simulink model "DFIG_DTC_1"  (R2014a)
settings: Solver=ode23tb  StartTime=0.0  StopTime=1  RelTol=1e-3
libraries: powerlib x11, powerlib_meascontrol x5, simulink x1
settings Model: Creator=ninad gaikawad  LastModifiedBy=ninad gaikawad
settings SolverCC: ZeroCrossAlgorithm=Adaptive

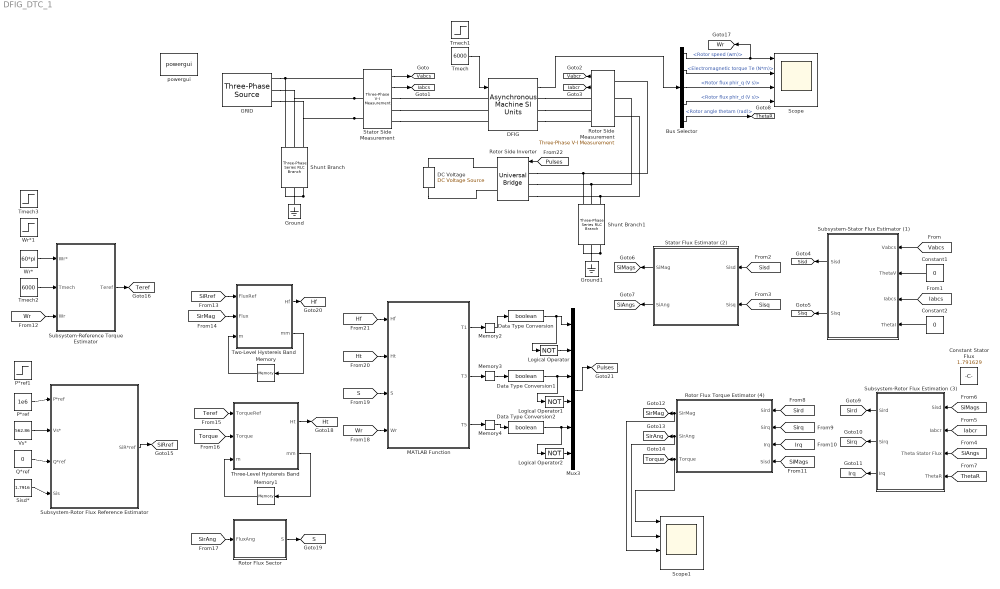
== system DFIG_DTC_1 ==
  Bus Selector : BusSelector  OutputSignals=Mechanical.Rotor speed (wm),Mechanical.Electromagnetic torque Te (N*m),Rotor measurements.Rotor flux phir_q (V s),Rotor measurements.Rotor flux phir_d (V s),Mechanical.Rotor angle thetam (rad)
  Constant Stator Flux : Constant  Value=1.791629
  Constant1 : Constant  Value=0
  Constant2 : Constant  Value=0
  DC Voltage : powerlib/Electrical Sources/DC Voltage Source  Amplitude=1200  Measurements=None
  DFIG : powerlib/Machines/Asynchronous Machine SI Units  PresetModel=No  MechanicalLoad=Torque Tm  ShowDetailedParameters=on  RotorType=Wound  ReferenceFrame=Rotor  Units=SI  MeasurementBus=off  NominalParameters=[1.5e+06 690 50]  Stator=[0.012 0.0137]  Rotor=[0.021 0.0136]  Cage1=[ 0.022 0.226/377]  Cage2=[ 0.022 0.226/377]  Lm=0.0135  Mechanical=[1000 30 2]  PolePairs=2  InitialConditions=[1 0 0 0 0 0 0 0]  SimulateSaturation=off  Saturation=[14.03593122, 27.81365428, 53.79336849, 72.68890987, 97.98006896, 148.6815601, 215.7428561, 302.9841135, 420.4778367 ; 230, 322, 414, 460, 506, 552, 598, 644, 690]  LoadFlowParameters=1492000  TsPowergui=0  TsBlock=-1  IterativeModel=Trapezoidal non iterative  Pmec=0
  Data Type Conversion : DataTypeConversion  OutDataTypeStr=boolean
  Data Type Conversion1 : DataTypeConversion  OutDataTypeStr=boolean
  Data Type Conversion2 : DataTypeConversion  OutDataTypeStr=boolean
  GRID : powerlib/Electrical Sources/Three-Phase Source  Voltage=25e3  PhaseAngle=0  Frequency=50  InternalConnection=Yg  SpecifyImpedance=off  Resistance=0  Inductance=0  ShortCircuitLevel=100e6  BaseVoltage=398  XRratio=7  BusType=swing  Pref=0  Qref=0  Qmin=-inf  Qmax=inf
  Ground : powerlib/Elements/Ground  LConnTagsString=a
  Ground1 : powerlib/Elements/Ground  LConnTagsString=a
  Logical Operator : Logic  Operator=NOT  AllPortsSameDT=off  OutDataTypeStr=boolean
  Logical Operator1 : Logic  Operator=NOT  AllPortsSameDT=off  OutDataTypeStr=boolean
  Logical Operator2 : Logic  Operator=NOT  AllPortsSameDT=off  OutDataTypeStr=boolean
  MATLAB Function : MATLAB Function  TreatAsAtomicUnit=on
  Memory : Memory  X0=1
  Memory1 : Memory  X0=1
  Memory2 : Memory  X0=1
  Memory3 : Memory
  Memory4 : Memory
  Mux3 : Mux  Inputs=6
  P*ref : Constant  Value=1e6
  P*ref1 : Step  Time=0.5  After=1e6  SampleTime=0
  Q*ref : Constant  Value=0
  Rotor Flux Sector : MATLAB Function  TreatAsAtomicUnit=on
  Rotor Flux Torque Estimator (4) : MATLAB Function  TreatAsAtomicUnit=on
  Rotor Side Inverter : powerlib/Power Electronics/Universal Bridge  Arms=3  SnubberResistance=1e5  SnubberCapacitance=inf  Device=IGBT / Diodes  Ron=1e-3  Lon=0  ForwardVoltages="[  0  0  ]"  ForwardVoltage=0  GTOparameters=[ 10e-6 , 20e-6 ]  IGBTparameters=[ 1e-6 , 2e-6 ]  Measurements=None  Measurements_2=None  converterType=Rectifier
  Rotor Side Measurement : powerlib/Measurements/Three-Phase V-I Measurement  VoltageMeasurement=phase-to-ground  SetLabelV=off  LabelV=Vabc  Vpu=off  VpuLL=off  CurrentMeasurement=yes  SetLabelI=off  LabelI=Iabc  Ipu=off  Pbase=100e6  Vbase=500e3  OutputType=Complex  PhasorSimulation=off  PSBequivalent=0
  Scope : Scope  NumInputPorts=4
      settings: YMin=-5~-5~-5~-5  YMax=5~5~5~5
  Scope1 : Scope  NumInputPorts=4
      settings: YMin=-5~-5~-5~-5  YMax=5~5~5~5
  Shunt Branch : powerlib/Elements/Three-Phase Series RLC Branch  LConnTagsString=A|B|C  RConnTagsString=A|B|C  BranchType=R  Resistance=1000  Inductance=1e-3  Capacitance=1e-6  Measurements=None
  Shunt Branch1 : powerlib/Elements/Three-Phase Series RLC Branch  LConnTagsString=A|B|C  RConnTagsString=A|B|C  BranchType=R  Resistance=10  Inductance=1e-3  Capacitance=1e-6  Measurements=None
  Sisd* : Constant  Value=1.7916
  Stator Flux Estimator (2) : MATLAB Function  TreatAsAtomicUnit=on
  Stator Side Measurement : powerlib/Measurements/Three-Phase V-I Measurement  VoltageMeasurement=phase-to-ground  SetLabelV=off  LabelV=Vabc  Vpu=off  VpuLL=off  CurrentMeasurement=yes  SetLabelI=off  LabelI=Iabc  Ipu=off  Pbase=100e6  Vbase=500e3  OutputType=Complex  PhasorSimulation=off  PSBequivalent=0
  Subsystem-Reference Torque Estimator : Subsystem
  Subsystem-Rotor Flux Estimation (3) : Subsystem
  Subsystem-Rotor Flux Reference Estimator : Subsystem
  Subsystem-Stator Flux Estimator (1) : Subsystem
  Three-Level Hystereis Band : MATLAB Function  TreatAsAtomicUnit=on
  Tmech : Constant  Value=6000
  Tmech1 : Step  Time=0.5  After=8000  SampleTime=0
  Tmech2 : Constant  Value=6000
  Tmech3 : Step  Time=0.5  After=8000  SampleTime=0
  Two-Level Hystereis Band : MATLAB Function  TreatAsAtomicUnit=on
  Vs* : Constant  Value=562.86
  Wr* : Constant  Value=60*pi
  Wr*1 : Step  Time=0.5  After=40*pi  SampleTime=0
  powergui : powerlib/powergui  Priority=1  SimulationMode=Continuous  SolverType=Tustin  SampleTime=50e-6  frequency=60  SPID=off  DisableSnubberDevices=off  DisableRonSwitches=off  DisableVfSwitches=off  SwTol=0  Interpol=off  DisplayEquations=off  Ts=0  methode=off  frequencyindice=50  Pbase=100e6  ErrMax=1e-4  Iterations=50  UnitsV=kV  UnitsW=MW  FunctionMessages=off  echomessages=off  HookPort=off  EnableUseOfTLC=off  x0status=blocks  RestoreLinks=warning  ResistiveCurrentMeasurement=off  Frange=[0:2:500]  Ylog=off  Xlog=on  ShowGrid=off  save=off  variable=ZData  structure=0  ZoomFFT=off  StartTime=0.0  cycles=1  DisplayStyle=1  fundamental=60  FreqAxis=off  MaxFrequency=1000  frequencyindicesteady=1  RmsSteady=1  display=off
  tag scope: Hf=global, Ht=global, Iabcr=global, Iabcs=global, Irq=global, Pulses=global, S=global, SiAngs=global, SiMags=global, SiRref=global, SirAng=global, SirMag=global, Sird=global, Sirq=global, Sisd=global, Sisq=global, Teref=global, ThetaR=global, Torque=global, Vabcr=global, Vabcs=global, Wr=global
  wires:
  DFIG/1 -> Bus Selector/1
  Stator Side Measurement/1 -> [Vabcs]
  Stator Side Measurement/2 -> [Iabcs]
  Rotor Side Measurement/1 -> [Vabcr]
  Rotor Side Measurement/2 -> [Iabcr]
  Bus Selector/2 -> Scope/2  "<Electromagnetic torque Te (N*m)>"
  Bus Selector/3 -> Scope/3  "<Rotor flux phir_q (V s)>"
  Bus Selector/4 -> Scope/4  "<Rotor flux phir_d (V s)>"
  Bus Selector/1 -> [Wr], Scope/1  "<Rotor speed (wm)>"
  [Vabcs] -> Subsystem-Stator Flux Estimator (1)/1(Vabcs)
  Constant1/1 -> Subsystem-Stator Flux Estimator (1)/2(ThetaV)
  [Iabcs] -> Subsystem-Stator Flux Estimator (1)/3(Iabcs)
  Constant2/1 -> Subsystem-Stator Flux Estimator (1)/4(ThetaI)
  Subsystem-Stator Flux Estimator (1)/1(Sisd) -> [Sisd]
  Subsystem-Stator Flux Estimator (1)/2(Sisq) -> [Sisq]
  [Sisd] -> Stator Flux Estimator (2)/1(Sisd)
  [Sisq] -> Stator Flux Estimator (2)/2(Sisq)
  Stator Flux Estimator (2)/2(SiAng) -> [SiAngs]
  Stator Flux Estimator (2)/1(SiMag) -> [SiMags]
  Bus Selector/5 -> [ThetaR]  "<Rotor angle thetam (rad)>"
  [SiMags] -> Subsystem-Rotor Flux Estimation (3)/1(Sisd)
  [Iabcr] -> Subsystem-Rotor Flux Estimation (3)/2(Iabcr)
  [SiAngs] -> Subsystem-Rotor Flux Estimation (3)/3(Theta Stator Flux)
  [ThetaR] -> Subsystem-Rotor Flux Estimation (3)/4(ThetaR)
  Subsystem-Rotor Flux Estimation (3)/2(Sirq) -> [Sirq]
  Subsystem-Rotor Flux Estimation (3)/1(Sird) -> [Sird]
  Subsystem-Rotor Flux Estimation (3)/3(Irq) -> [Irq]
  [SiMags] -> Rotor Flux Torque Estimator (4)/4(Sisd)
  [Irq] -> Rotor Flux Torque Estimator (4)/3(Irq)
  [Sirq] -> Rotor Flux Torque Estimator (4)/2(Sirq)
  [Sird] -> Rotor Flux Torque Estimator (4)/1(Sird)
  Rotor Flux Torque Estimator (4)/3(Torque) -> Scope1/1, [Torque]
  Q*ref/1 -> Subsystem-Rotor Flux Reference Estimator/3(Q*ref)
  Sisd*/1 -> Subsystem-Rotor Flux Reference Estimator/4(Sis)
  Subsystem-Rotor Flux Reference Estimator/1(SiR*ref) -> [SiRref]
  P*ref/1 -> Subsystem-Rotor Flux Reference Estimator/1(P*ref)
  Vs*/1 -> Subsystem-Rotor Flux Reference Estimator/2(Vs*)
  Tmech/1 -> DFIG/1
  Wr*/1 -> Subsystem-Reference Torque Estimator/1(Wr*)
  Subsystem-Reference Torque Estimator/1(Teref) -> [Teref]
  [Wr] -> Subsystem-Reference Torque Estimator/3(Wr)
  Tmech2/1 -> Subsystem-Reference Torque Estimator/2(Tmech)
  [SiRref] -> Two-Level Hystereis Band/1(FluxRef)
  [SirMag] -> Two-Level Hystereis Band/2(Flux)
  Two-Level Hystereis Band/2(mm) -> Memory/1
  Memory/1 -> Two-Level Hystereis Band/3(m)
  Three-Level Hystereis Band/2(mm) -> Memory1/1
  Memory1/1 -> Three-Level Hystereis Band/3(m)
  [Torque] -> Three-Level Hystereis Band/2(Torque)
  [Teref] -> Three-Level Hystereis Band/1(TorqueRef)
  [SirAng] -> Rotor Flux Sector/1(FluxAng)
  Rotor Flux Sector/1(S) -> [S]
  Three-Level Hystereis Band/1(Ht) -> [Ht]
  Two-Level Hystereis Band/1(Hf) -> [Hf]
  [Wr] -> MATLAB Function/4(Wr)
  Logical Operator1/1 -> Mux3/4
  Logical Operator/1 -> Mux3/2
  Logical Operator2/1 -> Mux3/6
  Data Type Conversion2/1 -> Logical Operator2/1, Mux3/5
  Data Type Conversion1/1 -> Logical Operator1/1, Mux3/3
  Memory2/1 -> Data Type Conversion/1
  MATLAB Function/1(T1) -> Memory2/1
  Memory3/1 -> Data Type Conversion1/1
  Memory4/1 -> Data Type Conversion2/1
  MATLAB Function/2(T3) -> Memory3/1
  MATLAB Function/3(T5) -> Memory4/1
  Data Type Conversion/1 -> Logical Operator/1, Mux3/1
  [Hf] -> MATLAB Function/1(Hf)
  [Ht] -> MATLAB Function/2(Ht)
  [S] -> MATLAB Function/3(S)
  Mux3/1 -> [Pulses]
  [Pulses] -> Rotor Side Inverter/1
  Rotor Flux Torque Estimator (4)/2(SirAng) -> Scope1/2, [SirAng]
  Rotor Flux Torque Estimator (4)/1(SirMag) -> Scope1/3, [SirMag]
  connections:
  GRID/RConn1 -- Stator Side Measurement/LConn1 -- Shunt Branch/LConn1
  Stator Side Measurement/LConn2 -- GRID/RConn2 -- Shunt Branch/LConn2
  Stator Side Measurement/LConn3 -- GRID/RConn3 -- Shunt Branch/LConn3
  Shunt Branch/RConn3 -- Shunt Branch/RConn1 -- Ground/LConn1 -- Shunt Branch/RConn2
  Rotor Side Inverter/LConn3 -- Shunt Branch1/LConn3 -- Rotor Side Measurement/LConn3
  DFIG/RConn2 -- Rotor Side Measurement/RConn2
  DFIG/RConn3 -- Rotor Side Measurement/RConn3
  Stator Side Measurement/RConn2 -- DFIG/LConn2
  Stator Side Measurement/RConn3 -- DFIG/LConn3
  Stator Side Measurement/RConn1 -- DFIG/LConn1
  DC Voltage/RConn1 -- Rotor Side Inverter/RConn1
  DC Voltage/LConn1 -- Rotor Side Inverter/RConn2
  DFIG/RConn1 -- Rotor Side Measurement/RConn1
  Rotor Side Inverter/LConn2 -- Shunt Branch1/LConn2 -- Rotor Side Measurement/LConn2
  Rotor Side Inverter/LConn1 -- Shunt Branch1/LConn1 -- Rotor Side Measurement/LConn1
  Shunt Branch1/RConn3 -- Shunt Branch1/RConn1 -- Ground1/LConn1 -- Shunt Branch1/RConn2

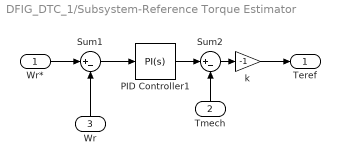
== system DFIG_DTC_1/Subsystem-Reference Torque Estimator ==
  Wr* : Inport
  Tmech : Inport  Port=2
  Wr : Inport  Port=3
  PID Controller1 : simulink/Continuous/PID Controller  Controller=PI  TimeDomain=Continuous-time  SampleTime=1  IntegratorMethod=Forward Euler  FilterMethod=Forward Euler  Form=Parallel  P=273.240186106265  I=55.6628456867696  D=0  N=100  InitialConditionSource=internal  InitialConditionForIntegrator=0  InitialConditionForFilter=0  ExternalReset=none  LimitOutput=off  UpperSaturationLimit=inf  LowerSaturationLimit=-inf  LinearizeAsGain=on  AntiWindupMode=none  Kb=1  TrackingMode=off  Kt=1  PParamMin=[]  PParamMax=[]  IParamMin=[]  IParamMax=[]  DParamMin=[]  DParamMax=[]  NParamMin=[]  NParamMax=[]  KbParamMin=[]  KbParamMax=[]  KtParamMin=[]  KtParamMax=[]  POutMin=[]  POutMax=[]  IOutMin=[]  IOutMax=[]  DOutMin=[]  DOutMax=[]  NOutMin=[]  NOutMax=[]  KbOutMin=[]  KbOutMax=[]  KtOutMin=[]  KtOutMax=[]  IntegratorOutMin=[]  IntegratorOutMax=[]  FilterOutMin=[]  FilterOutMax=[]  SumOutMin=[]  SumOutMax=[]  SumI1OutMin=[]  SumI1OutMax=[]  SumI2OutMin=[]  SumI2OutMax=[]  SumI3OutMin=[]  SumI3OutMax=[]  SumDOutMin=[]  SumDOutMax=[]  SaturationOutMin=[]  SaturationOutMax=[]  IntegratorContinuousStateAttributes=''  IntegratorStateMustResolveToSignalObject=off  IntegratorRTWStateStorageClass=Auto  FilterContinuousStateAttributes=''  FilterStateMustResolveToSignalObject=off  FilterRTWStateStorageClass=Auto
  Sum1 : Sum  Inputs=|+-
  Sum2 : Sum  Inputs=|+-
  k : Gain  Gain=-1
  Teref : Outport
  wires:
  Wr/1 -> Sum1/2
  Sum1/1 -> PID Controller1/1
  Tmech/1 -> Sum2/2
  PID Controller1/1 -> Sum2/1
  k/1 -> Teref/1
  Sum2/1 -> k/1
  Wr*/1 -> Sum1/1

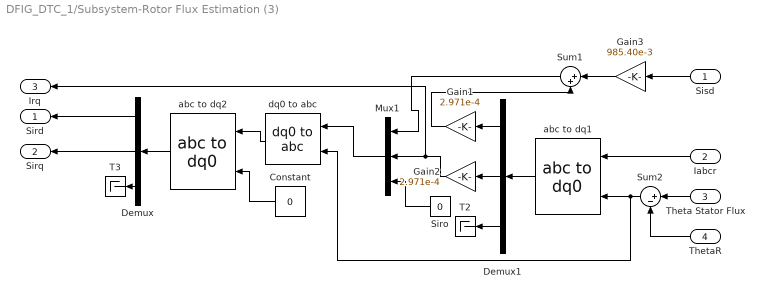
== system DFIG_DTC_1/Subsystem-Rotor Flux Estimation (3) ==
  Sisd : Inport
  Iabcr : Inport  Port=2
  Theta Stator Flux : Inport  Port=3
  ThetaR : Inport  Port=4
  Constant : Constant  Value=0
  Demux : Demux  Outputs=3
  Demux1 : Demux  Outputs=3
  Gain1 : Gain  Gain=2.971e-4
  Gain2 : Gain  Gain=2.971e-4
  Gain3 : Gain  Gain=985.40e-3
  Mux1 : Mux  Inputs=3
  Siro : Constant  Value=0
  Sum1 : Sum  Inputs=|++
  Sum2 : Sum  Inputs=|+-
  T2 : Terminator
  T3 : Terminator
  abc to dq1 : powerlib_meascontrol/Transformations/abc to dq0  Alignment=Aligned with phase A axis
  abc to dq2 : powerlib_meascontrol/Transformations/abc to dq0  Alignment=Aligned with phase A axis
  dq0 to abc : powerlib_meascontrol/Transformations/dq0 to abc  Alignment=Aligned with phase A axis
  Sird : Outport
  Sirq : Outport  Port=2
  Irq : Outport  Port=3
  wires:
  Sum1/1 -> Mux1/1
  Demux/3 -> T3/1
  Demux/2 -> Sirq/1
  Siro/1 -> Mux1/3
  Demux/1 -> Sird/1
  Iabcr/1 -> abc to dq1/1
  Gain1/1 -> Sum1/2
  Theta Stator Flux/1 -> Sum2/1
  Constant/1 -> abc to dq2/2
  Sum2/1 -> dq0 to abc/2, abc to dq1/2
  dq0 to abc/1 -> abc to dq2/1
  abc to dq2/1 -> Demux/1
  ThetaR/1 -> Sum2/2
  Demux1/1 -> Gain1/1
  Demux1/3 -> T2/1
  Demux1/2 -> Gain2/1
  abc to dq1/1 -> Demux1/1
  Mux1/1 -> dq0 to abc/1
  Gain2/1 -> Irq/1, Mux1/2
  Sisd/1 -> Gain3/1
  Gain3/1 -> Sum1/1

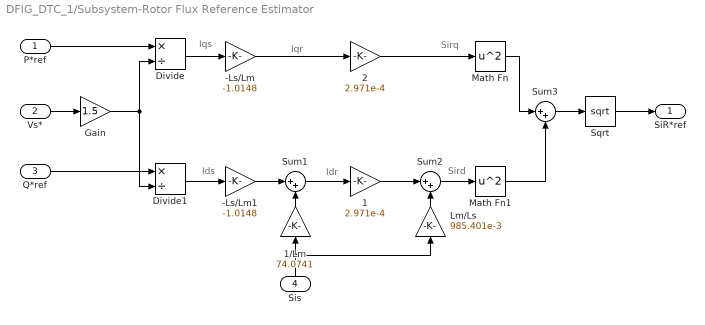
== system DFIG_DTC_1/Subsystem-Rotor Flux Reference Estimator ==
  note: Sird
  note: Sirq
  note: Ids
  note: Iqs
  note: Idr
  note: Iqr
  P*ref : Inport
  Vs* : Inport  Port=2
  Q*ref : Inport  Port=3
  Sis : Inport  Port=4
  -Ls/Lm : Gain  Gain=-1.0148
  -Ls/Lm1 : Gain  Gain=-1.0148
  1 : Gain  Gain=2.971e-4
  1/Lm : Gain  Gain=74.0741
  2 : Gain  Gain=2.971e-4
  Divide : Product  Inputs=*/
  Divide1 : Product  Inputs=*/
  Gain : Gain  Gain=1.5
  Lm/Ls : Gain  Gain=985.401e-3
  Math Fn : Math  Operator=square  SaturateOnIntegerOverflow=on
  Math Fn1 : Math  Operator=square  SaturateOnIntegerOverflow=on
  Sqrt : Sqrt  SaturateOnIntegerOverflow=on
  Sum1 : Sum  Inputs=|++
  Sum2 : Sum  Inputs=|++
  Sum3 : Sum  Inputs=|++
  SiR*ref : Outport
  wires:
  P*ref/1 -> Divide/1
  Vs*/1 -> Gain/1
  Q*ref/1 -> Divide1/1
  Divide/1 -> -Ls/Lm/1
  -Ls/Lm1/1 -> Sum1/1
  Sis/1 -> Lm/Ls/1, 1/Lm/1
  Divide1/1 -> -Ls/Lm1/1
  1/Lm/1 -> Sum1/2
  Gain/1 -> Divide1/2, Divide/2
  Sqrt/1 -> SiR*ref/1
  2/1 -> Math Fn/1
  1/1 -> Sum2/1
  Sum2/1 -> Math Fn1/1
  Sum1/1 -> 1/1
  -Ls/Lm/1 -> 2/1
  Math Fn1/1 -> Sum3/2
  Sum3/1 -> Sqrt/1
  Math Fn/1 -> Sum3/1
  Lm/Ls/1 -> Sum2/2

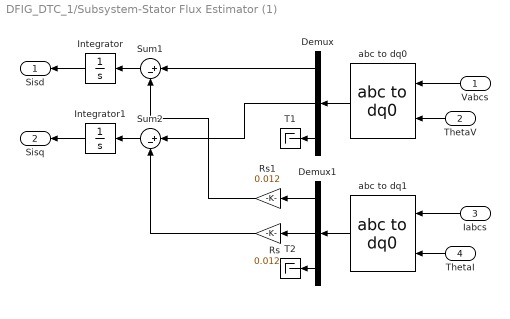
== system DFIG_DTC_1/Subsystem-Stator Flux Estimator (1) ==
  Vabcs : Inport
  ThetaV : Inport  Port=2
  Iabcs : Inport  Port=3
  ThetaI : Inport  Port=4
  Demux : Demux  Outputs=3
  Demux1 : Demux  Outputs=3
  Integrator : Integrator
  Integrator1 : Integrator
  Rs : Gain  Gain=0.012
  Rs1 : Gain  Gain=0.012
  Sum1 : Sum  Inputs=|+-
  Sum2 : Sum  Inputs=|+-
  T1 : Terminator
  T2 : Terminator
  abc to dq0 : powerlib_meascontrol/Transformations/abc to dq0  Alignment=Aligned with phase A axis
  abc to dq1 : powerlib_meascontrol/Transformations/abc to dq0  Alignment=Aligned with phase A axis
  Sisd : Outport
  Sisq : Outport  Port=2
  wires:
  Sum2/1 -> Integrator1/1
  Sum1/1 -> Integrator/1
  abc to dq0/1 -> Demux/1
  ThetaI/1 -> abc to dq1/2
  Iabcs/1 -> abc to dq1/1
  Rs1/1 -> Sum1/2
  Demux1/3 -> T2/1
  abc to dq1/1 -> Demux1/1
  Vabcs/1 -> abc to dq0/1
  Demux/1 -> Sum1/1
  Rs/1 -> Sum2/2
  Demux/3 -> T1/1
  Demux1/2 -> Rs/1
  Demux1/1 -> Rs1/1
  Demux/2 -> Sum2/1
  ThetaV/1 -> abc to dq0/2
  Integrator/1 -> Sisd/1
  Integrator1/1 -> Sisq/1

== matlab function DFIG_DTC_1/Two-Level Hystereis Band ==
  data: FluxRef input; Hf output; Flux input; m input; mm output
function [Hf,mm] = Two_Level_Hys(FluxRef,Flux,m)
 
DelF=0.025;% Hysteresis Width for Flux
Hf=0;%Initializing Hysteresis Controller Output For Flux
mm=m;
% Flux Two Level Hysteresis Band %
%------------------------------------------------------------------------%
if(Flux<=(FluxRef-DelF))
    Hf=1;
    mm=Hf;
end
if(mm==1&&(Flux>(FluxRef-DelF))&&(Flux<(FluxRef+DelF)))
    Hf=1;
    mm=Hf;
end
if(Flux>=(FluxRef+DelF))
    Hf=0;
    mm=Hf;
end
if(mm==0&&(Flux>(FluxRef-DelF))&&(Flux<(FluxRef+DelF)))
    Hf=0;
    mm=Hf;
end

== matlab function DFIG_DTC_1/Rotor Flux Torque Estimator (4) ==
  data: Sird input; SirMag output; Sirq input; Irq input; Sisd input; SirAng output; Torque output
function [SirMag,SirAng,Torque] = Rotor_Flux_Torque_Estimator(Sird,Sirq,Irq,Sisd)
 SirMag=((Sird)^(2)+(Sirq)^(2))^(0.5);
 x=atan2(Sirq,Sird);
 if(x>=0)
    SirAng=x*(180/pi);
 else
    SirAng=x*(180/pi)+360;
 end
 Torque=(-3)*(0.0135/0.0136)*(Sisd*Irq);

== matlab function DFIG_DTC_1/Stator Flux Estimator (2) ==
  settings: updateMethod=CONTINUOUS
  data: Sisd input; SiMag output; Sisq input; SiAng output
function [SiMag,SiAng] = StatorFlux_MagAng_Estimator(Sisd,Sisq)
 SiMag=((Sisd)^(2)+(Sisq)^(2))^(0.5);
 x=atan2(Sisq,Sisd);
 if(x>=0)
    SiAng=x;
 else
    SiAng=x+(2*pi);
 end

== matlab function DFIG_DTC_1/Three-Level Hystereis Band ==
  data: TorqueRef input; Ht output; Torque input; m input; mm output
function [Ht,mm] = Three_Level_Hys(TorqueRef,Torque,m)
 
DelT=1;% Hysteresis Width for Torque
Ht=0;%Initializing Hysteresis Controller Output For Torque
mm=m;

% Torque Three Level Hysteresis Band %
%------------------------------------------------------------------------%
if(Torque<=(TorqueRef-DelT))
    Ht=1;
    mm=Ht;
end
if((Torque>(TorqueRef-DelT))&&(Torque<TorqueRef)&&mm==1)
    Ht=1;
    mm=Ht;
end
if(Torque>=(TorqueRef+DelT))
    Ht=-1;
    mm=Ht;
end
if((Torque<(TorqueRef+DelT))&&(Torque>TorqueRef)&&mm==-1)
    Ht=-1;
    mm=Ht;
end
if((Torque>(TorqueRef-DelT))&&(Torque<TorqueRef)&&mm==-1)
    Ht=0;
    mm=-1;
end
if((Torque<(TorqueRef+DelT))&&(Torque>TorqueRef)&&mm==1)
    Ht=0;
    mm=1;
end

== matlab function DFIG_DTC_1/Rotor Flux Sector ==
  data: FluxAng input; S output
function S= Rotor_Flux_Sector(FluxAng)
 

% DTC Sector Prediction %
%------------------------------------------------------------------------%
if(FluxAng>=330&&FluxAng<30)
    S=1;
end
if(FluxAng>=30&&FluxAng<90)
    S=2;
end
if(FluxAng>=90&&FluxAng<150)
    S=3;
end
if(FluxAng>=150&&FluxAng<210)
    S=4;
end
if(FluxAng>=210&&FluxAng<270)
    S=5;
end
if(FluxAng>=270&&FluxAng<330)
    S=6;
end

== matlab function DFIG_DTC_1/MATLAB Function ==
  data: Hf input; T1 output; Ht input; S input; Wr input; T3 output; T5 output
function [T1,T3,T5] = DTC_SwitchingTable(Hf,Ht,S,Wr)
 
T1=0;
T3=0;
T5=0;

% Voltage Vector Synthesis %
%------------------------------------------------------------------------%
if(Wr<=(50*pi))% Sub-Synchronous
%------------------------------------------------------------------------%    
    if(Hf==1&&Ht==1&&S==1)
        T1=1;
        T3=0;
        T5=1;
    end
    if(Hf==1&&Ht==1&&S==2)
      T1=0;
      T3=0;
      T5=1;  
    end
    if(Hf==1&&Ht==1&&S==3)
      T1=0;
      T3=1;
      T5=1; 
    end
    if(Hf==1&&Ht==1&&S==4)
      T1=0;
      T3=1;
      T5=0;
    end
    if(Hf==1&&Ht==1&&S==5)
      T1=1;
      T3=1;
      T5=0;    
    end
    if(Hf==1&&Ht==1&&S==6)
      T1=1;
      T3=0;
      T5=0;
    end
   
%------------------------------------------------------------------------%    
    if(Hf==1&&Ht==0&&S==1)
        T1=1;
        T3=1;
        T5=1;
    end
    if(Hf==1&&Ht==0&&S==2)
      T1=0;
      T3=0;
      T5=0;  
    end
    if(Hf==1&&Ht==0&&S==3)
      T1=1;
      T3=1;
      T5=1; 
    end
    if(Hf==1&&Ht==0&&S==4)
      T1=0;
      T3=0;
      T5=0;
    end
    if(Hf==1&&Ht==0&&S==5)
      T1=1;
      T3=1;
      T5=1;    
    end
    if(Hf==1&&Ht==0&&S==6)
      T1=0;
      T3=0;
      T5=0;
    end
%------------------------------------------------------------------------%    
    if(Hf==1&&Ht==-1&&S==1)
        T1=1;
        T3=1;
        T5=0;
    end
    if(Hf==1&&Ht==-1&&S==2)
      T1=1;
      T3=0;
      T5=0;  
    end
    if(Hf==1&&Ht==-1&&S==3)
      T1=1;
      T3=0;
      T5=1; 
    end
    if(Hf==1&&Ht==-1&&S==4)
      T1=0;
      T3=0;
      T5=1;
    end
    if(Hf==1&&Ht==-1&&S==5)
      T1=0;
      T3=1;
      T5=1;    
    end
    if(Hf==1&&Ht==-1&&S==6)
      T1=0;
      T3=1;
      T5=0;
    end
    
 %------------------------------------------------------------------------%   
    
     if(Hf==0&&Ht==1&&S==1)
        T1=0;
        T3=0;
        T5=1;
    end
    if(Hf==0&&Ht==1&&S==2)
      T1=0;
      T3=1;
      T5=1;  
    end
    if(Hf==0&&Ht==1&&S==3)
      T1=0;
      T3=1;
      T5=0; 
    end
    if(Hf==0&&Ht==1&&S==4)
      T1=1;
      T3=1;
      T5=0;
    end
    if(Hf==0&&Ht==1&&S==5)
      T1=1;
      T3=0;
      T5=0;    
    end
    if(Hf==0&&Ht==1&&S==6)
      T1=1;
      T3=0;
      T5=1;
    end
%------------------------------------------------------------------------%    
    
    if(Hf==0&&Ht==0&&S==1)
        T1=0;
        T3=0;
        T5=0;
    end
    if(Hf==0&&Ht==0&&S==2)
      T1=1;
      T3=1;
      T5=1;  
    end
    if(Hf==0&&Ht==0&&S==3)
      T1=0;
      T3=0;
      T5=0; 
    end
    if(Hf==0&&Ht==0&&S==4)
      T1=1;
      T3=1;
      T5=1;
    end
    if(Hf==0&&Ht==0&&S==5)
      T1=0;
      T3=0;
      T5=0;    
    end
    if(Hf==0&&Ht==0&&S==6)
      T1=1;
      T3=1;
      T5=1;
    end
  %------------------------------------------------------------------------%  
    
    if(Hf==0&&Ht==-1&&S==1)
        T1=0;
        T3=1;
        T5=0;
    end
    if(Hf==0&&Ht==-1&&S==2)
      T1=1;
      T3=1;
      T5=0;  
    end
    if(Hf==0&&Ht==-1&&S==3)
      T1=1;
      T3=0;
      T5=0; 
    end
    if(Hf==0&&Ht==-1&&S==4)
      T1=1;
      T3=0;
      T5=1;
    end
    if(Hf==0&&Ht==-1&&S==5)
      T1=0;
      T3=0;
      T5=1;    
    end
    if(Hf==0&&Ht==-1&&S==6)
      T1=0;
      T3=1;
      T5=1;
    end
end

%------------------------------------------------------------------------%
if(Wr>(50*pi))% Super-Synchronous
%------------------------------------------------------------------------%    
    if(Hf==1&&Ht==1&&S==1)
        T1=1;
        T3=0;
        T5=1;
    end
    if(Hf==1&&Ht==1&&S==2)
      T1=1;
      T3=0;
      T5=0;  
    end
    if(Hf==1&&Ht==1&&S==3)
      T1=1;
      T3=1;
      T5=0; 
    end
    if(Hf==1&&Ht==1&&S==4)
      T1=0;
      T3=1;
      T5=0;
    end
    if(Hf==1&&Ht==1&&S==5)
      T1=0;
      T3=1;
      T5=1;    
    end
    if(Hf==1&&Ht==1&&S==6)
      T1=0;
      T3=0;
      T5=1;
    end
   
%------------------------------------------------------------------------%    
    if(Hf==1&&Ht==0&&S==1)
        T1=1;
        T3=1;
        T5=1;
    end
    if(Hf==1&&Ht==0&&S==2)
      T1=0;
      T3=0;
      T5=0;  
    end
    if(Hf==1&&Ht==0&&S==3)
      T1=1;
      T3=1;
      T5=1; 
    end
    if(Hf==1&&Ht==0&&S==4)
      T1=0;
      T3=0;
      T5=0;
    end
    if(Hf==1&&Ht==0&&S==5)
      T1=1;
      T3=1;
      T5=1;    
    end
    if(Hf==1&&Ht==0&&S==6)
      T1=0;
      T3=0;
      T5=0;
    end
%------------------------------------------------------------------------%    
    if(Hf==1&&Ht==-1&&S==1)
        T1=1;
        T3=0;
        T5=0;
    end
    if(Hf==1&&Ht==-1&&S==2)
      T1=1;
      T3=1;
      T5=0;  
    end
    if(Hf==1&&Ht==-1&&S==3)
      T1=0;
      T3=1;
      T5=0; 
    end
    if(Hf==1&&Ht==-1&&S==4)
      T1=0;
      T3=1;
      T5=1;
    end
    if(Hf==1&&Ht==-1&&S==5)
      T1=0;
      T3=0;
      T5=1;    
    end
    if(Hf==1&&Ht==-1&&S==6)
      T1=1;
      T3=0;
      T5=1;
    end
    
 %------------------------------------------------------------------------%   
    
     if(Hf==0&&Ht==1&&S==1)
        T1=0;
        T3=0;
        T5=1;
    end
    if(Hf==0&&Ht==1&&S==2)
      T1=1;
      T3=0;
      T5=1;  
    end
    if(Hf==0&&Ht==1&&S==3)
      T1=1;
      T3=0;
      T5=0; 
    end
    if(Hf==0&&Ht==1&&S==4)
      T1=1;
      T3=1;
      T5=0;
    end
    if(Hf==0&&Ht==1&&S==5)
      T1=0;
      T3=1;
      T5=0;    
    end
    if(Hf==0&&Ht==1&&S==6)
      T1=0;
      T3=1;
      T5=1;
    end
%------------------------------------------------------------------------%    
    
    if(Hf==0&&Ht==0&&S==1)
        T1=0;
        T3=0;
        T5=0;
    end
    if(Hf==0&&Ht==0&&S==2)
      T1=1;
      T3=1;
      T5=1;  
    end
    if(Hf==0&&Ht==0&&S==3)
      T1=0;
      T3=0;
      T5=0; 
    end
    if(Hf==0&&Ht==0&&S==4)
      T1=1;
      T3=1;
      T5=1;
    end
    if(Hf==0&&Ht==0&&S==5)
      T1=0;
      T3=0;
      T5=0;    
    end
    if(Hf==0&&Ht==0&&S==6)
      T1=1;
      T3=1;
      T5=1;
    end
  %------------------------------------------------------------------------%  
    
    if(Hf==0&&Ht==-1&&S==1)
        T1=0;
        T3=1;
        T5=1;
    end
    if(Hf==0&&Ht==-1&&S==2)
      T1=0;
      T3=0;
      T5=1;  
    end
    if(Hf==0&&Ht==-1&&S==3)
      T1=1;
      T3=0;
      T5=1; 
    end
    if(Hf==0&&Ht==-1&&S==4)
      T1=1;
      T3=0;
      T5=0;
    end
    if(Hf==0&&Ht==-1&&S==5)
      T1=1;
      T3=1;
      T5=0;    
    end
    if(Hf==0&&Ht==-1&&S==6)
      T1=0;
      T3=1;
      T5=0;
    end
end
